simulink model "Example"  (R2020b)
settings: Solver=VariableStepAuto  StartTime=0.0  StopTime=10.0  RelTol=1e-3
settings Model: Creator=riwakaram  LastModifiedBy=riwakaram

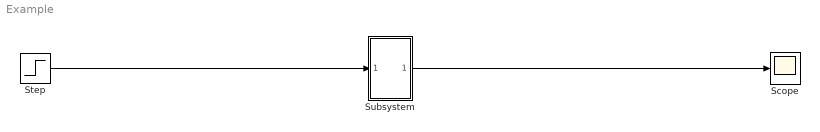
== system Example ==
  Scope : Scope
  Step : Step  SampleTime=0
  Subsystem : Subsystem
  wires:
  Step/1 -> Subsystem/1(In1)
  Subsystem/1(Out1) -> Scope/1

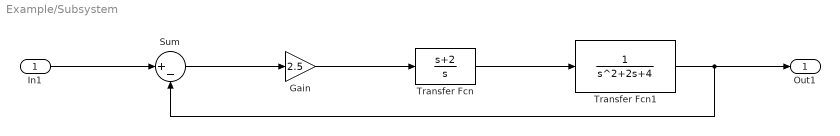
== system Example/Subsystem ==
  In1 : Inport
  Gain : Gain  Gain=2.5
  Sum : Sum  Inputs=|+-
  Transfer Fcn : TransferFcn  Numerator=[1 2]  Denominator=[1 0]
  Transfer Fcn1 : TransferFcn  Denominator=[1 2 4]
  Out1 : Outport
  wires:
  In1/1 -> Sum/1
  Gain/1 -> Transfer Fcn/1
  Transfer Fcn1/1 -> Out1/1, Sum/2
  Sum/1 -> Gain/1
  Transfer Fcn/1 -> Transfer Fcn1/1
